simulink model "simplified_model"  (R2019b)
settings: Solver=VariableStepAuto  StartTime=0.0  StopTime=10.0  RelTol=1e-3
values from neighbouring files (symbols this model uses):
  K_d = [10 0; 0 10]    [parameters.m]
  K_p = [25 0; 0 25]    [parameters.m]
settings Model: Creator=stephhan  LastModifiedBy=stephhan

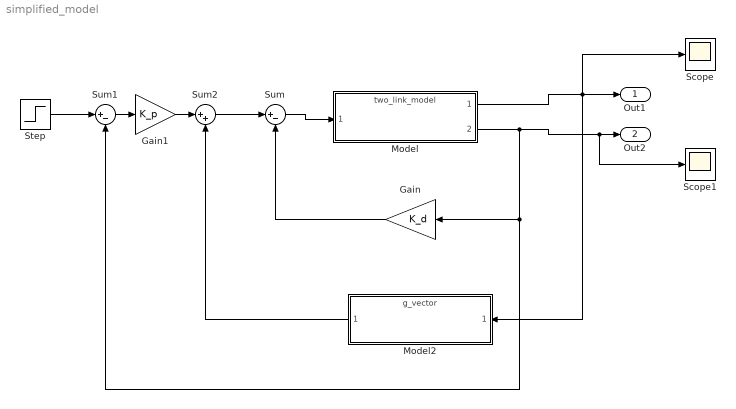
== system simplified_model ==
  Gain : Gain  Gain=K_d
  Gain1 : Gain  Gain=K_p
  Model : ModelReference  ModelNameDialog=two_link_model  SimulationMode=Normal  ModelReferenceVersion=1.3
  Model2 : ModelReference  ModelNameDialog=g_vector.slx  SimulationMode=Normal  ModelReferenceVersion=1.8
  Scope : Scope
  Scope1 : Scope
  Step : Step  SampleTime=0
  Sum : Sum  Inputs=|+-
  Sum1 : Sum  Inputs=|+-
  Sum2 : Sum  Inputs=|++
  Out1 : Outport
  Out2 : Outport  Port=2
  wires:
  Sum1/1 -> Gain1/1
  Gain1/1 -> Sum2/1
  Model/1 -> Scope/1, Model2/1, Out1/1
  Model/2 -> Sum1/2, Gain/1, Scope1/1, Out2/1
  Sum2/1 -> Sum/1
  Sum/1 -> Model/1
  Gain/1 -> Sum/2
  Step/1 -> Sum1/1
  Model2/1 -> Sum2/2
